simulink library "THAMO_6x2"  (R2018a)
settings: Solver=VariableStepAuto  StartTime=0.0  StopTime=10.0  RelTol=1e-3
undefined symbols (not defined in the file): BM, DiameterLastPiece, DPConstant, DPLinear, DPQuadratic, GeodeticHeight, ID, magnitude, MassFlow, Pressure, Temperature, Water
libraries: carnot x11, simulink x10, $bdroot x3
(part 3 of 3)

== system THAMO_6x2/Ventil/pressuredrop ==
  mdot : Inport
  p_in : Inport  Port=2
  clq_in : Inport  Port=3
  qua : Inport  Port=4
  Constant : Constant
  Constant1 : Constant  Value=0
  Constant2 : Constant  Value=0
  Dot Product : DotProduct  InputSameDT=on  OutDataTypeStr=Inherit: Inherit via internal rule
  Math Function : Math  Operator=square  SaturateOnIntegerOverflow=on
  Mux : Mux  Inputs=3
  Mux1 : Mux  Inputs=3
  Saturation : Saturate  UpperLimit=inf  LowerLimit=0
  sum : Sum  SaturateOnIntegerOverflow=on  InputSameDT=on  OutDataTypeStr=Inherit: Same as first input
  sum1 : Sum  Inputs=+-  SaturateOnIntegerOverflow=on  InputSameDT=on  OutDataTypeStr=Inherit: Same as first input
  p_out : Outport
  clq_out : Outport  Port=2
  wires:
  Saturation/1 -> p_out/1
  Constant/1 -> Mux/1
  mdot/1 -> Mux/2, Math Function/1
  Math Function/1 -> Mux/3
  Mux/1 -> Dot Product/1
  qua/1 -> Mux1/3
  clq_in/1 -> sum/1
  sum/1 -> clq_out/1
  Mux1/1 -> sum/2, Dot Product/2
  Dot Product/1 -> sum1/2
  p_in/1 -> sum1/1
  sum1/1 -> Saturation/1
  Constant1/1 -> Mux1/1
  Constant2/1 -> Mux1/2

== system THAMO_6x2/Verbraucher_RK-Modell/HK_MST_Ruehrkesselkask ==
  THB__1_W : Inport
  t__L : Inport  Port=2
  Bus Selector : BusSelector  OutputSignals=Temperature,MassFlow
  Bus Selector1 : BusSelector  OutputSignals=Temperature
  Constant1 : Constant  Value=t_1N
  Constant2 : Constant  Value=20
  Constant3 : Constant  Value=t_2N
  Mux : Mux  Inputs=3
  Subsystem : Subsystem
  THB_set_T : carnot/Source/Simple/THB_set_T
  cp : Lookup_n-D  NumberOfTableDimensions=1  BreakpointsForDimension1=[0,10,20,30,40,50,60,70,80,90,100]  Table=[4218,4192,4182,4179,4179,4181,4184,4190,4196,4205,4216]  InternalRulePriority=Speed  RndMeth=Simplest  InputSameDT=on
  dtlogN : Fcn  Expr=(u(1)-u(2))/log((u(1)-u(3))/(u(2)-u(3)))
  THB__2_W : Outport
  Qdot_2 : Outport  Port=2
  wires:
  Bus Selector1/1 -> cp/1  "<Temperature>"
  cp/1 -> Subsystem/4(cp)
  Subsystem/2(Qdot_he_w) -> Qdot_2/1  "Q_MST"
  Subsystem/1(T_he_out) -> THB_set_T/2  "T_RL_MST"
  dtlogN/1 -> Subsystem/5(dTlogN)
  THB__1_W/1 -> THB_set_T/1, Bus Selector/1, Bus Selector1/1
  THB_set_T/1 -> THB__2_W/1
  Bus Selector/2 -> Subsystem/2(mdot_w)  "<MassFlow>"
  Bus Selector/1 -> Subsystem/1(T_he_in)  "<Temperature>"
  t__L/1 -> Subsystem/3(T_i)
  Constant1/1 -> Mux/1
  Constant3/1 -> Mux/2
  Constant2/1 -> Mux/3
  Mux/1 -> dtlogN/1

== system THAMO_6x2/Verbraucher_RK-Modell/Pressure_Drop ==
  THB__1_W : Inport
  Bus Assignment1 : BusAssignment  AssignedSignals=Pressure,DPConstant,DPLinear,DPQuadratic
  Bus Selector3 : BusSelector  OutputSignals=MassFlow,Pressure
  Bus Selector4 : BusSelector  OutputSignals=DPConstant,DPLinear,DPQuadratic  OutputAsBus=on
  Bus Selector5 : BusSelector  OutputSignals=ID
  Compare To Constant1 : simulink/Logic and Bit Operations/Compare To Constant  relop=>  const=0  OutDataTypeStr=boolean
  Demux2 : Demux  Outputs=3
  Pressuredrop : carnot/Basic/Pressure_Drop/Pressuredrop
  lq_calc : Subsystem
  THB__2_W : Outport
  wires:
  Compare To Constant1/1 -> lq_calc/Enable
  lq_calc/1(qua) -> Pressuredrop/4
  Demux2/3 -> Bus Assignment1/5
  Demux2/2 -> Bus Assignment1/4
  Demux2/1 -> Bus Assignment1/3
  Bus Assignment1/1 -> THB__2_W/1
  Pressuredrop/1 -> Bus Assignment1/2
  THB__1_W/1 -> Bus Selector5/1, lq_calc/1(THB__1_W), Bus Selector4/1, Bus Selector3/1, Bus Assignment1/1
  Bus Selector4/1 -> Pressuredrop/3
  Bus Selector3/1 -> Pressuredrop/1  "<MassFlow>"
  Bus Selector3/2 -> Pressuredrop/2  "<Pressure>"
  Bus Selector5/1 -> Compare To Constant1/1  "<ID>"
  Pressuredrop/2 -> Demux2/1

== system THAMO_6x2/Wärmeabnehmer/Pressure_Drop ==
  THB__1_W : Inport
  Bus Assignment1 : BusAssignment  AssignedSignals=Pressure,DPConstant,DPLinear,DPQuadratic
  Bus Selector3 : BusSelector  OutputSignals=MassFlow,Pressure
  Bus Selector4 : BusSelector  OutputSignals=DPConstant,DPLinear,DPQuadratic  OutputAsBus=on
  Bus Selector5 : BusSelector  OutputSignals=ID
  Compare To Constant1 : simulink/Logic and Bit Operations/Compare To Constant  relop=>  const=0  OutDataTypeStr=boolean
  Demux2 : Demux  Outputs=3
  Pressuredrop : Subsystem  mask(pressure drop){}
      mask help:
      | Pressure drop according to input values of con, lin and qua:
      | dp = con + lin*mdot + qua*mdot²
      | The coefficients are also added to the correponding THB elements.
      mask Help: web(fullfile(path_carnot('help'),'Pressuredrop.html'),'-helpbrowser')
  lq_calc : Subsystem
  THB__2_W : Outport
  wires:
  Compare To Constant1/1 -> lq_calc/Enable
  lq_calc/1(qua) -> Pressuredrop/4(qua)
  Demux2/3 -> Bus Assignment1/5
  Demux2/2 -> Bus Assignment1/4
  Demux2/1 -> Bus Assignment1/3
  Bus Assignment1/1 -> THB__2_W/1
  Pressuredrop/1(p_out) -> Bus Assignment1/2
  THB__1_W/1 -> Bus Selector5/1, lq_calc/1(THB__1_W), Bus Selector4/1, Bus Selector3/1, Bus Assignment1/1
  Bus Selector4/1 -> Pressuredrop/3(clq_in)
  Bus Selector3/1 -> Pressuredrop/1(mdot)  "<MassFlow>"
  Bus Selector3/2 -> Pressuredrop/2(p_in)  "<Pressure>"
  Bus Selector5/1 -> Compare To Constant1/1  "<ID>"
  Pressuredrop/2(clq_out) -> Demux2/1

== system THAMO_6x2/Wärmeabnehmer/Temperatur ==
  THB__1_W : Inport
  Qdot_2 : Inport  Port=2
  Bus Assignment : BusAssignment  AssignedSignals=Temperature
  Bus Selector : BusSelector  OutputSignals=Temperature,MassFlow
  Fcn : Fcn  Expr=u(1)-u(4)/u(3)/u(2)
  Mux : Mux
  Thermal_Capacity : Subsystem  mask(Thermal Capacity){}
      mask help: Basic one node model of a thermal mass using the differential equation:
      mask Help: web(fullfile(path_carnot('help'),'Thermal_Capacity.html'),'-helpbrowser')
  cp_W : Lookup_n-D  NumberOfTableDimensions=1  BreakpointsForDimension1=[0,10,20,30,40,50,60,70,80,90,100]  Table=[4218,4192,4182,4179,4179,4181,4184,4190,4196,4205,4216]  InternalRulePriority=Speed  RndMeth=Simplest  InputSameDT=on
  THB__2_W : Outport
  wires:
  THB__1_W/1 -> Bus Assignment/1, Bus Selector/1
  Bus Assignment/1 -> Thermal_Capacity/1(THB__1_W)
  cp_W/1 -> Mux/3
  Bus Selector/2 -> Mux/2  "<MassFlow>"
  Bus Selector/1 -> cp_W/1, Mux/1  "<Temperature>"
  Qdot_2/1 -> Mux/4
  Mux/1 -> Fcn/1
  Fcn/1 -> Bus Assignment/2
  Thermal_Capacity/1(THB__2_W) -> THB__2_W/1

== system THAMO_6x2/Wärmeerzeuger/Pressure_Drop ==
  THB__1_W : Inport
  Bus Assignment1 : BusAssignment  AssignedSignals=Pressure,DPConstant,DPLinear,DPQuadratic
  Bus Selector3 : BusSelector  OutputSignals=MassFlow,Pressure
  Bus Selector4 : BusSelector  OutputSignals=DPConstant,DPLinear,DPQuadratic  OutputAsBus=on
  Bus Selector5 : BusSelector  OutputSignals=ID
  Compare To Constant1 : simulink/Logic and Bit Operations/Compare To Constant  relop=>  const=0  OutDataTypeStr=boolean
  Demux2 : Demux  Outputs=3
  Pressuredrop : carnot/Basic/Pressure_Drop/Pressuredrop
  lq_calc : Subsystem
  THB__2_W : Outport
  wires:
  Compare To Constant1/1 -> lq_calc/Enable
  lq_calc/1(qua) -> Pressuredrop/4
  Demux2/3 -> Bus Assignment1/5
  Demux2/2 -> Bus Assignment1/4
  Demux2/1 -> Bus Assignment1/3
  Bus Assignment1/1 -> THB__2_W/1
  Pressuredrop/1 -> Bus Assignment1/2
  THB__1_W/1 -> Bus Selector5/1, lq_calc/1(THB__1_W), Bus Selector4/1, Bus Selector3/1, Bus Assignment1/1
  Bus Selector4/1 -> Pressuredrop/3
  Bus Selector3/1 -> Pressuredrop/1  "<MassFlow>"
  Bus Selector3/2 -> Pressuredrop/2  "<Pressure>"
  Bus Selector5/1 -> Compare To Constant1/1  "<ID>"
  Pressuredrop/2 -> Demux2/1

== system THAMO_6x2/Wärmeerzeuger/Thermal_Capacity ==
  mdot : Inport
  Tin : Inport  Port=2
  Divide : Product  Inputs=*/
  Integrator : Integrator  InitialCondition=Tamb
  Losses : Gain  Gain=UV  SaturateOnIntegerOverflow=on  OutDataTypeStr=Inherit: Same as input  ParamDataTypeStr=Inherit: Same as input
  Product1 : Product  Inputs=3  SaturateOnIntegerOverflow=on  InputSameDT=on  OutDataTypeStr=Inherit: Same as first input
  Product3 : Product  Inputs=3  SaturateOnIntegerOverflow=on  InputSameDT=on  OutDataTypeStr=Inherit: Same as first input
  Sum1 : Sum  Inputs=-+  SaturateOnIntegerOverflow=on  InputSameDT=on  OutDataTypeStr=Inherit: Same as first input
  Sum2 : Sum  Inputs=-+  SaturateOnIntegerOverflow=on  InputSameDT=on  OutDataTypeStr=Inherit: Same as first input
  Sum3 : Sum  Inputs=+-  SaturateOnIntegerOverflow=on  InputSameDT=on  OutDataTypeStr=Inherit: Same as first input
  Tamb : Constant  Value=Tamb
  Tamb1 : Constant  Value=V/1000
  cp : Lookup_n-D  NumberOfTableDimensions=1  BreakpointsForDimension1=[0,10,20,30,40,50,60,70,80,90,100]  Table=[4218,4192,4182,4179,4179,4181,4184,4190,4196,4205,4216]  InternalRulePriority=Speed  RndMeth=Simplest  InputSameDT=on
  rho : Lookup_n-D  NumberOfTableDimensions=1  BreakpointsForDimension1=[0,10,20,30,40,50,60,70,80,90,100]  Table=[999.84,999.7,998.2,995.64,992.21,988.03,983.19,977.76,971.79,965.3,958.35]  InternalRulePriority=Speed  RndMeth=Simplest  InputSameDT=on
  Tout : Outport
  wires:
  mdot/1 -> Product1/2
  Product1/1 -> Sum2/2
  Sum2/1 -> Divide/1
  Tamb/1 -> Sum3/2
  Losses/1 -> Sum2/1
  Sum3/1 -> Losses/1
  cp/1 -> Product3/1, Product1/3
  Divide/1 -> Integrator/1
  Sum1/1 -> Product1/1
  Tin/1 -> Sum1/2
  Product3/1 -> Divide/2
  rho/1 -> Product3/2
  Tamb1/1 -> Product3/3
  Integrator/1 -> rho/1, cp/1, Sum1/1, Sum3/1, Tout/1

== system THAMO_6x2/Überströmventil/pressuredrop ==
  mdot : Inport
  p_in : Inport  Port=2
  clq_in : Inport  Port=3
  con : Inport  Port=4
  lin : Inport  Port=5
  qua : Inport  Port=6
  Constant : Constant
  Dot Product : DotProduct  InputSameDT=on  OutDataTypeStr=Inherit: Inherit via internal rule
  Math Function : Math  Operator=square  SaturateOnIntegerOverflow=on
  Mux : Mux  Inputs=3
  Mux1 : Mux  Inputs=3
  Saturation : Saturate  UpperLimit=inf  LowerLimit=0
  sum : Sum  SaturateOnIntegerOverflow=on  InputSameDT=on  OutDataTypeStr=Inherit: Same as first input
  sum1 : Sum  Inputs=+-  SaturateOnIntegerOverflow=on  InputSameDT=on  OutDataTypeStr=Inherit: Same as first input
  p_out : Outport
  clq_out : Outport  Port=2
  wires:
  lin/1 -> Mux1/2
  con/1 -> Mux1/1
  sum1/1 -> Saturation/1
  p_in/1 -> sum1/1
  Dot Product/1 -> sum1/2
  Mux1/1 -> Dot Product/2, sum/2
  sum/1 -> clq_out/1
  clq_in/1 -> sum/1
  qua/1 -> Mux1/3
  Mux/1 -> Dot Product/1
  Math Function/1 -> Mux/3
  mdot/1 -> Math Function/1, Mux/2
  Constant/1 -> Mux/1
  Saturation/1 -> p_out/1

== system THAMO_6x2/Brennwertkessel/Combustion_Calculation/cp___A ==
  eco : Inport
  Add : Sum  Inputs=+++++++
  Add1 : Sum  Inputs=+++++++
  Bus Selector1 : BusSelector  OutputSignals=mdotH20,mdotCO2,mdot_O2,mdotSO2,mdotN2,mdotNOx,mdot_CO
  Divide : Product  Inputs=/*
  Product{,1..6} (7 alike) : Product
  cpCO : Constant  Value=1.04
  cpCO2 : Constant  Value=0.846
  cpH2O : Constant  Value=1.85
  cpN2 : Constant  Value=1.04
  cpNOx : Constant  Value=1.009
  cpO2 : Constant  Value=0.912
  cpSO2 : Constant  Value=0.632
  cp___A : Outport
  wires:
  Add/1 -> Divide/1
  Add1/1 -> Divide/2
  Divide/1 -> cp___A/1
  Product1/1 -> Add1/2
  Product2/1 -> Add1/3
  Product3/1 -> Add1/4
  Product4/1 -> Add1/5
  Product5/1 -> Add1/6
  Product/1 -> Add1/1
  Product6/1 -> Add1/7
  cpCO2/1 -> Product1/2
  cpO2/1 -> Product2/2
  cpSO2/1 -> Product3/2
  cpN2/1 -> Product4/2
  cpNOx/1 -> Product5/2
  cpCO/1 -> Product6/2
  cpH2O/1 -> Product/2
  Bus Selector1/7 -> Add/7, Product6/1  "<mdot_CO>"
  Bus Selector1/1 -> Add/1, Product/1  "<mdotH20>"
  Bus Selector1/2 -> Add/2, Product1/1  "<mdotCO2>"
  Bus Selector1/3 -> Add/3, Product2/1  "<mdot_O2>"
  Bus Selector1/4 -> Add/4, Product3/1  "<mdotSO2>"
  Bus Selector1/6 -> Add/6, Product5/1  "<mdotNOx>"
  Bus Selector1/5 -> Add/5, Product4/1  "<mdotN2>"
  eco/1 -> Bus Selector1/1

== system THAMO_6x2/Brennwertkessel/Combustion_Calculation/exhaust gas ==
  h : Inport
  c : Inport  Port=2
  s : Inport  Port=3
  n : Inport  Port=4
  w : Inport  Port=5
  Mux : Mux  Inputs=2
  kgCO2 : Gain  Gain=44.01/12  SaturateOnIntegerOverflow=on  OutDataTypeStr=Inherit: Same as input  ParamDataTypeStr=Inherit: Same as input
  kgH2O : Fcn  Expr=(18.01/1.008/2)*u(1)+u(2)
  kgN2 : Gain  Gain=0.5  SaturateOnIntegerOverflow=on  OutDataTypeStr=Inherit: Same as input  ParamDataTypeStr=Inherit: Same as input
  kgSO2 : Gain  Gain=64.06/32.06  SaturateOnIntegerOverflow=on  OutDataTypeStr=Inherit: Same as input  ParamDataTypeStr=Inherit: Same as input
  H2O : Outport
  CO2 : Outport  Port=2
  SO2 : Outport  Port=3
  N2 : Outport  Port=4
  wires:
  n/1 -> kgN2/1
  kgSO2/1 -> SO2/1
  kgH2O/1 -> H2O/1
  kgCO2/1 -> CO2/1
  Mux/1 -> kgH2O/1
  c/1 -> kgCO2/1
  h/1 -> Mux/1
  w/1 -> Mux/2
  s/1 -> kgSO2/1
  kgN2/1 -> N2/1

== system THAMO_6x2/Brennwertkessel/Pressure_Drop/lq_calc ==
  THB__1_W : Inport
  Enable : EnablePort
  Bus Selector1 : BusSelector  OutputSignals=Temperature,MassFlow
  Constant : Constant  Value=BM
  Constant1 : Constant  Value=kvs
  Constant2 : Constant  Value=zeta
  Constant3 : Constant  Value=d
  Constant4 : Constant  Value=m_N
  Constant5 : Constant  Value=dp_N
  Multiport Switch : MultiPortSwitch
  Mux : Mux  Inputs=2
  Mux1 : Mux  Inputs=2
  Mux2 : Mux
  calc_qua_N : Fcn  Expr=u(2)/u(1)^2
  calc_qua_kvs : Fcn  Expr=(3600^2*100)/(u(1)^2*u(2))
  calc_qua_zeta : Fcn  Expr=(((u(3)/u(1))/(3.1415/4*(u(4)/1000)^2))^2*u(2)*u(1)/2)/u(3)^2
  rho : Lookup_n-D  NumberOfTableDimensions=1  BreakpointsForDimension1=[0,10,20,30,40,50,60,70,80,90,100]  Table=[999.84,999.7,998.2,995.64,992.21,988.03,983.19,977.76,971.79,965.3,958.35]  InternalRulePriority=Speed  RndMeth=Simplest  InputSameDT=on
  qua : Outport
  wires:
  calc_qua_zeta/1 -> Multiport Switch/3
  Constant2/1 -> Mux2/2
  Mux2/1 -> calc_qua_zeta/1
  Bus Selector1/2 -> Mux2/3  "<MassFlow>"
  Constant3/1 -> Mux2/4
  calc_qua_N/1 -> Multiport Switch/4
  Constant5/1 -> Mux1/2
  Constant4/1 -> Mux1/1
  Mux1/1 -> calc_qua_N/1
  calc_qua_kvs/1 -> Multiport Switch/2
  Mux/1 -> calc_qua_kvs/1
  rho/1 -> Mux/2, Mux2/1
  Constant1/1 -> Mux/1
  Constant/1 -> Multiport Switch/1
  Multiport Switch/1 -> qua/1
  THB__1_W/1 -> Bus Selector1/1
  Bus Selector1/1 -> rho/1  "<Temperature>"

== system THAMO_6x2/Mischer/Ventil/Ventilkennlinie ==
  St : Inport
  THB__1_W : Inport  Port=2
  Bus Selector : BusSelector  OutputSignals=Temperature
  Constant2 : Constant  Value=ART
  Constant6 : Constant  Value=n_0
  Constant8 : Constant  Value=kvs
  GLP : Fcn  Expr=u(2)*((1/u(2))^u(1))
  Mux : Mux  Inputs=2
  Mux2 : Mux  Inputs=2
  Mux3 : Mux  Inputs=2
  Product : Product
  Switch : Switch  Criteria=u2 > Threshold  Threshold=1
  calc_qua_kvs : Fcn  Expr=(3600^2*100)/(u(1)^2*u(2))
  linear : Fcn  Expr=u(2)+(1-u(2))*u(1)
  rho : Lookup_n-D  NumberOfTableDimensions=1  BreakpointsForDimension1=[0,10,20,30,40,50,60,70,80,90,100]  Table=[999.84,999.7,998.2,995.64,992.21,988.03,983.19,977.76,971.79,965.3,958.35]  InternalRulePriority=Speed  RndMeth=Simplest  InputSameDT=on
  qua : Outport
  wires:
  rho/1 -> Mux/2
  Product/1 -> Mux/1
  Mux/1 -> calc_qua_kvs/1
  calc_qua_kvs/1 -> qua/1
  THB__1_W/1 -> Bus Selector/1
  GLP/1 -> Switch/1
  Constant2/1 -> Switch/2
  Switch/1 -> Product/1
  Constant8/1 -> Product/2
  Constant6/1 -> Mux3/2, Mux2/2
  Mux3/1 -> linear/1
  Mux2/1 -> GLP/1
  linear/1 -> Switch/3
  St/1 -> Mux3/1, Mux2/1
  Bus Selector/1 -> rho/1  "<Temperature>"

== system THAMO_6x2/Mischer/Ventil/pressuredrop ==
  mdot : Inport
  p_in : Inport  Port=2
  clq_in : Inport  Port=3
  qua : Inport  Port=4
  Constant : Constant
  Constant1 : Constant  Value=0
  Constant2 : Constant  Value=0
  Dot Product : DotProduct  InputSameDT=on  OutDataTypeStr=Inherit: Inherit via internal rule
  Math Function : Math  Operator=square  SaturateOnIntegerOverflow=on
  Mux : Mux  Inputs=3
  Mux1 : Mux  Inputs=3
  Saturation : Saturate  UpperLimit=inf  LowerLimit=0
  sum : Sum  SaturateOnIntegerOverflow=on  InputSameDT=on  OutDataTypeStr=Inherit: Same as first input
  sum1 : Sum  Inputs=+-  SaturateOnIntegerOverflow=on  InputSameDT=on  OutDataTypeStr=Inherit: Same as first input
  p_out : Outport
  clq_out : Outport  Port=2
  wires:
  Constant2/1 -> Mux1/2
  Constant1/1 -> Mux1/1
  sum1/1 -> Saturation/1
  p_in/1 -> sum1/1
  Dot Product/1 -> sum1/2
  Mux1/1 -> Dot Product/2, sum/2
  sum/1 -> clq_out/1
  clq_in/1 -> sum/1
  qua/1 -> Mux1/3
  Mux/1 -> Dot Product/1
  Math Function/1 -> Mux/3
  mdot/1 -> Math Function/1, Mux/2
  Constant/1 -> Mux/1
  Saturation/1 -> p_out/1

== system THAMO_6x2/Mischer/Ventil1/Ventilkennlinie ==
  St : Inport
  THB__1_W : Inport  Port=2
  Bus Selector : BusSelector  OutputSignals=Temperature
  Constant2 : Constant  Value=ART
  Constant6 : Constant  Value=n_0
  Constant8 : Constant  Value=kvs
  GLP : Fcn  Expr=u(2)*((1/u(2))^u(1))
  Mux : Mux  Inputs=2
  Mux2 : Mux  Inputs=2
  Mux3 : Mux  Inputs=2
  Product : Product
  Switch : Switch  Criteria=u2 > Threshold  Threshold=1
  calc_qua_kvs : Fcn  Expr=(3600^2*100)/(u(1)^2*u(2))
  linear : Fcn  Expr=u(2)+(1-u(2))*u(1)
  rho : Lookup_n-D  NumberOfTableDimensions=1  BreakpointsForDimension1=[0,10,20,30,40,50,60,70,80,90,100]  Table=[999.84,999.7,998.2,995.64,992.21,988.03,983.19,977.76,971.79,965.3,958.35]  InternalRulePriority=Speed  RndMeth=Simplest  InputSameDT=on
  qua : Outport
  wires:
  rho/1 -> Mux/2
  Product/1 -> Mux/1
  Mux/1 -> calc_qua_kvs/1
  calc_qua_kvs/1 -> qua/1
  THB__1_W/1 -> Bus Selector/1
  GLP/1 -> Switch/1
  Constant2/1 -> Switch/2
  Switch/1 -> Product/1
  Constant8/1 -> Product/2
  Constant6/1 -> Mux3/2, Mux2/2
  Mux3/1 -> linear/1
  Mux2/1 -> GLP/1
  linear/1 -> Switch/3
  St/1 -> Mux3/1, Mux2/1
  Bus Selector/1 -> rho/1  "<Temperature>"

== system THAMO_6x2/Mischer/Ventil1/pressuredrop ==
  mdot : Inport
  p_in : Inport  Port=2
  clq_in : Inport  Port=3
  qua : Inport  Port=4
  Constant : Constant
  Constant1 : Constant  Value=0
  Constant2 : Constant  Value=0
  Dot Product : DotProduct  InputSameDT=on  OutDataTypeStr=Inherit: Inherit via internal rule
  Math Function : Math  Operator=square  SaturateOnIntegerOverflow=on
  Mux : Mux  Inputs=3
  Mux1 : Mux  Inputs=3
  Saturation : Saturate  UpperLimit=inf  LowerLimit=0
  sum : Sum  SaturateOnIntegerOverflow=on  InputSameDT=on  OutDataTypeStr=Inherit: Same as first input
  sum1 : Sum  Inputs=+-  SaturateOnIntegerOverflow=on  InputSameDT=on  OutDataTypeStr=Inherit: Same as first input
  p_out : Outport
  clq_out : Outport  Port=2
  wires:
  Constant2/1 -> Mux1/2
  Constant1/1 -> Mux1/1
  sum1/1 -> Saturation/1
  p_in/1 -> sum1/1
  Dot Product/1 -> sum1/2
  Mux1/1 -> Dot Product/2, sum/2
  sum/1 -> clq_out/1
  clq_in/1 -> sum/1
  qua/1 -> Mux1/3
  Mux/1 -> Dot Product/1
  Math Function/1 -> Mux/3
  mdot/1 -> Math Function/1, Mux/2
  Constant/1 -> Mux/1
  Saturation/1 -> p_out/1

== system THAMO_6x2/Rohr/Druckverlust/Pressuredrop ==
  mdot : Inport
  p_in : Inport  Port=2
  clq_in : Inport  Port=3
  con : Inport  Port=4
  lin : Inport  Port=5
  qua : Inport  Port=6
  Constant : Constant
  Dot Product : DotProduct  InputSameDT=on  OutDataTypeStr=Inherit: Inherit via internal rule
  Math Function : Math  Operator=square  SaturateOnIntegerOverflow=on
  Mux : Mux  Inputs=3
  Mux1 : Mux  Inputs=3
  Saturation : Saturate  UpperLimit=inf  LowerLimit=0
  sum : Sum  SaturateOnIntegerOverflow=on  InputSameDT=on  OutDataTypeStr=Inherit: Same as first input
  sum1 : Sum  Inputs=+-  SaturateOnIntegerOverflow=on  InputSameDT=on  OutDataTypeStr=Inherit: Same as first input
  p_out : Outport
  clq_out : Outport  Port=2
  wires:
  Saturation/1 -> p_out/1
  Constant/1 -> Mux/1
  mdot/1 -> Mux/2, Math Function/1
  Math Function/1 -> Mux/3
  Mux/1 -> Dot Product/1
  con/1 -> Mux1/1
  lin/1 -> Mux1/2
  qua/1 -> Mux1/3
  clq_in/1 -> sum/1
  sum/1 -> clq_out/1
  Mux1/1 -> sum/2, Dot Product/2
  Dot Product/1 -> sum1/2
  p_in/1 -> sum1/1
  sum1/1 -> Saturation/1

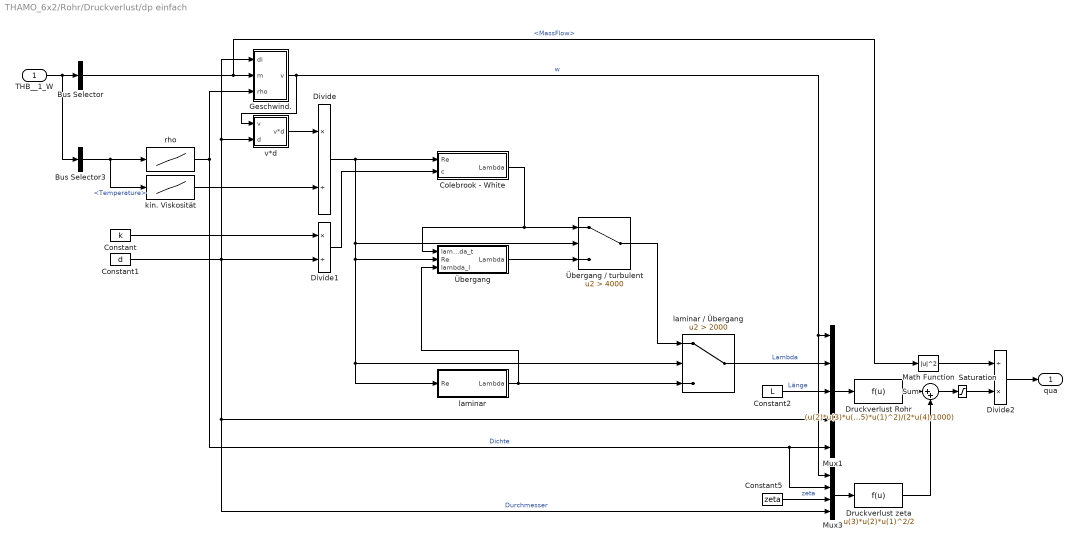
== system THAMO_6x2/Rohr/Druckverlust/dp einfach ==
  THB__1_W : Inport
  Bus Selector : BusSelector  OutputSignals=MassFlow
  Bus Selector3 : BusSelector  OutputSignals=Temperature
  Colebrook - White : Subsystem
  Constant : Constant  Value=k
  Constant1 : Constant  Value=d
  Constant2 : Constant  Value=L
  Constant5 : Constant  Value=zeta
  Divide : Product  Inputs=*/
  Divide1 : Product  Inputs=*/
  Divide2 : Product  Inputs=/*
  Druckverlust Rohr : Fcn  Expr=(u(2)*u(3)*u(5)*u(1)^2)/(2*u(4)/1000)
  Druckverlust zeta : Fcn  Expr=u(3)*u(2)*u(1)^2/2
  Geschwind. : Subsystem
  Math Function : Math  Operator=magnitude^2  SaturateOnIntegerOverflow=on
  Mux1 : Mux  Inputs=5
  Mux3 : Mux
  Saturation : Saturate  UpperLimit=inf  LowerLimit=1
  Sum : Sum  Inputs=|++
  kin. Viskosität : Lookup_n-D  NumberOfTableDimensions=1  BreakpointsForDimension1=[1,10,20,30,40,50,60,70,80,90,99]  Table=[0.017307,0.013061,0.010033,0.0080078,0.0065808,0.0055346,0.0047437,0.0041308,0.0036464,0.0032572,0.0029690]/(100*100)  InternalRulePriority=Speed  RndMeth=Simplest  InputSameDT=on
  laminar : Subsystem
  laminar / Übergang : Switch  Criteria=u2 > Threshold  Threshold=2000
  rho : Lookup_n-D  NumberOfTableDimensions=1  BreakpointsForDimension1=[0,10,20,30,40,50,60,70,80,90,100]  Table=[999.84,999.7,998.2,995.64,992.21,988.03,983.19,977.76,971.79,965.3,958.35]  InternalRulePriority=Speed  RndMeth=Simplest  InputSameDT=on
  v*d : Subsystem
  Übergang : Subsystem
  Übergang / turbulent : Switch  Criteria=u2 > Threshold  Threshold=4000
  qua : Outport
  wires:
  v*d/1(v*d) -> Divide/1
  Constant/1 -> Divide1/1
  Divide1/1 -> Colebrook - White/2(c)
  laminar/1(Lambda) -> laminar / Übergang/3, Übergang/3(lambda_l)
  laminar / Übergang/1 -> Mux1/2  "Lambda"
  Constant2/1 -> Mux1/3  "Länge"
  Mux1/1 -> Druckverlust Rohr/1
  rho/1 -> Geschwind./3(rho), Mux3/2, Mux1/5  "Dichte"
  Geschwind./1(v) -> Mux3/1, Mux1/1, v*d/1(v)  "w"
  Divide/1 -> Übergang / turbulent/2, Übergang/2(Re), laminar/1(Re), laminar / Übergang/2, Colebrook - White/1(Re)
  THB__1_W/1 -> Bus Selector3/1, Bus Selector/1
  Übergang / turbulent/1 -> laminar / Übergang/1
  Colebrook - White/1(Lambda) -> Übergang / turbulent/1, Übergang/1(lambda_t)
  Übergang/1(Lambda) -> Übergang / turbulent/3
  Constant1/1 -> Mux3/4, Mux1/4, v*d/2(d), Geschwind./1(di), Divide1/2  "Durchmesser"
  Mux3/1 -> Druckverlust zeta/1
  Constant5/1 -> Mux3/3  "zeta"
  Bus Selector/1 -> Math Function/1, Geschwind./2(m)  "<MassFlow>"
  Druckverlust Rohr/1 -> Sum/1
  Druckverlust zeta/1 -> Sum/2
  Math Function/1 -> Divide2/1
  Sum/1 -> Saturation/1
  Divide2/1 -> qua/1
  Saturation/1 -> Divide2/2
  Bus Selector3/1 -> kin. Viskosität/1, rho/1  "<Temperature>"
  kin. Viskosität/1 -> Divide/2

== system THAMO_6x2/T-Stueck mischend/Mixer/Mix_T_Mdot ==
  THB1 : Inport
  THB2 : Inport  Port=2
  Bus Selector1 : BusSelector  OutputSignals=MassFlow,Temperature
  Bus Selector2 : BusSelector  OutputSignals=MassFlow,Temperature
  Fcn : Fcn  Expr=(u(1)*u(2)+u(3)*u(4))/(u(1)+u(3))
  Mux : Mux
  T : Outport
  wires:
  THB2/1 -> Bus Selector1/1
  THB1/1 -> Bus Selector2/1
  Bus Selector2/2 -> Mux/2  "<Temperature>"
  Bus Selector2/1 -> Mux/1  "<MassFlow>"
  Bus Selector1/1 -> Mux/3  "<MassFlow>"
  Bus Selector1/2 -> Mux/4  "<Temperature>"
  Mux/1 -> Fcn/1
  Fcn/1 -> T/1

== system THAMO_6x2/T-Stueck mischend/Mixer/decrease_ID1 ==
  In1 : Inport
  Abs : Abs
  Bias : Bias  Bias=-1
  Dot Product1 : DotProduct  InputSameDT=on  OutDataTypeStr=Inherit: Inherit via internal rule
  Sign : Signum
  Out1 : Outport
  wires:
  Bias/1 -> Dot Product1/2
  Sign/1 -> Dot Product1/1
  Abs/1 -> Bias/1
  Dot Product1/1 -> Out1/1
  In1/1 -> Sign/1, Abs/1

== system THAMO_6x2/T-Stueck mischend/Mixer/decrease_ID2 ==
  In1 : Inport
  Abs : Abs
  Bias : Bias  Bias=-1
  Dot Product1 : DotProduct  InputSameDT=on  OutDataTypeStr=Inherit: Inherit via internal rule
  Sign : Signum
  Out1 : Outport
  wires:
  In1/1 -> Abs/1, Sign/1
  Dot Product1/1 -> Out1/1
  Abs/1 -> Bias/1
  Sign/1 -> Dot Product1/1
  Bias/1 -> Dot Product1/2

== system THAMO_6x2/Verbraucher_RK-Modell/HK_MST_Ruehrkesselkask/Subsystem ==
  T_he_in : Inport
  mdot_w : Inport  Port=2
  T_i : Inport  Port=3
  cp : Inport  Port=4
  dTlogN : Inport  Port=5
  Constant1 : Constant  Value=Qdot_N
  Constant2 : Constant  Value=n
  K : Fcn  Expr=u(3)/(u(1)^n)
  Mux : Mux  Inputs=6
  Mux1 : Mux  Inputs=6
  Mux2 : Mux  Inputs=6
  Mux3 : Mux
  Mux4 : Mux  Inputs=3
  Qdot_he_w_ : Fcn  Expr=u(4)*u(2)*(u(1)-u(3))
  T_w1 : Integrator  InitialConditionSource=external
  T_w2 : Integrator  InitialConditionSource=external
  T_w3 : Integrator  InitialConditionSource=external
  dT_w1/dt : Fcn  Expr=(3*u(2)*u(5)*(u(3)-u(1))-u(6)*(u(1)-u(4))^n)/(M*u(5))
  dT_w2/dt : Fcn  Expr=(3*u(2)*u(5)*(u(3)-u(1))-u(6)*(u(1)-u(4))^n)/(M*u(5))
  dT_w3/dt : Fcn  Expr=(3*u(2)*u(5)*(u(3)-u(1))-u(6)*(u(1)-u(4))^n)/(M*u(5))
  T_he_out : Outport
  Qdot_he_w : Outport  Port=2
  wires:
  K/1 -> Mux1/6, Mux/6, Mux2/6
  cp/1 -> Mux/5, Mux1/5, Mux2/5, Mux3/4  "cp"
  Mux4/1 -> K/1
  Constant1/1 -> Mux4/3
  Constant2/1 -> Mux4/2
  dTlogN/1 -> Mux4/1
  Mux2/1 -> dT_w3/dt/1
  Mux3/1 -> Qdot_he_w_/1
  Mux1/1 -> dT_w2/dt/1
  Mux/1 -> dT_w1/dt/1
  T_w2/1 -> Mux2/3, Mux1/1
  T_he_in/1 -> Mux/3, Mux3/1  "T_VL"
  dT_w2/dt/1 -> T_w2/1
  Qdot_he_w_/1 -> Qdot_he_w/1
  T_w3/1 -> Mux2/1, Mux3/3, T_he_out/1  "T_RL"
  T_i/1 -> Mux/4, T_w1/2, Mux1/4, Mux2/4, T_w3/2, T_w2/2
  T_w1/1 -> Mux1/3, Mux/1
  dT_w3/dt/1 -> T_w3/1
  dT_w1/dt/1 -> T_w1/1
  mdot_w/1 -> Mux3/2, Mux/2, Mux1/2, Mux2/2  "mdot"

== system THAMO_6x2/Verbraucher_RK-Modell/Pressure_Drop/lq_calc ==
  THB__1_W : Inport
  Enable : EnablePort
  Bus Selector : BusSelector  OutputSignals=MassFlow
  Bus Selector1 : BusSelector  OutputSignals=Temperature
  Constant : Constant  Value=BM
  Constant1 : Constant  Value=kvs
  Constant2 : Constant  Value=zeta
  Constant3 : Constant  Value=d
  Constant4 : Constant  Value=m_N
  Constant5 : Constant  Value=dp_N
  Multiport Switch : MultiPortSwitch
  Mux : Mux  Inputs=2
  Mux1 : Mux  Inputs=2
  Mux2 : Mux
  calc_qua_N : Fcn  Expr=u(2)/u(1)^2
  calc_qua_kvs : Fcn  Expr=(3600^2*100)/(u(1)^2*u(2))
  calc_qua_zeta : Fcn  Expr=(((u(3)/u(1))/(3.1415/4*(u(4)/1000)^2))^2*u(2)*u(1)/2)/u(3)^2
  rho : Lookup_n-D  NumberOfTableDimensions=1  BreakpointsForDimension1=[0,10,20,30,40,50,60,70,80,90,100]  Table=[999.84,999.7,998.2,995.64,992.21,988.03,983.19,977.76,971.79,965.3,958.35]  InternalRulePriority=Speed  RndMeth=Simplest  InputSameDT=on
  qua : Outport
  wires:
  Bus Selector1/1 -> rho/1  "<Temperature>"
  calc_qua_zeta/1 -> Multiport Switch/3
  Constant2/1 -> Mux2/2
  Mux2/1 -> calc_qua_zeta/1
  Bus Selector/1 -> Mux2/3  "<MassFlow>"
  Constant3/1 -> Mux2/4
  calc_qua_N/1 -> Multiport Switch/4
  Constant5/1 -> Mux1/2
  Constant4/1 -> Mux1/1
  Mux1/1 -> calc_qua_N/1
  calc_qua_kvs/1 -> Multiport Switch/2
  Mux/1 -> calc_qua_kvs/1
  rho/1 -> Mux/2, Mux2/1
  Constant1/1 -> Mux/1
  Constant/1 -> Multiport Switch/1
  Multiport Switch/1 -> qua/1
  THB__1_W/1 -> Bus Selector/1, Bus Selector1/1

== system THAMO_6x2/Wärmeabnehmer/Pressure_Drop/Pressuredrop ==
  mdot : Inport
  p_in : Inport  Port=2
  clq_in : Inport  Port=3
  qua : Inport  Port=4
  Constant : Constant
  Constant1 : Constant  Value=0
  Constant2 : Constant  Value=0
  Dot Product : DotProduct  InputSameDT=on  OutDataTypeStr=Inherit: Inherit via internal rule
  Math Function : Math  Operator=square  SaturateOnIntegerOverflow=on
  Mux : Mux  Inputs=3
  Mux1 : Mux  Inputs=3
  Saturation : Saturate  UpperLimit=inf  LowerLimit=0
  sum : Sum  SaturateOnIntegerOverflow=on  InputSameDT=on  OutDataTypeStr=Inherit: Same as first input
  sum1 : Sum  Inputs=+-  SaturateOnIntegerOverflow=on  InputSameDT=on  OutDataTypeStr=Inherit: Same as first input
  p_out : Outport
  clq_out : Outport  Port=2
  wires:
  Saturation/1 -> p_out/1
  Constant/1 -> Mux/1
  mdot/1 -> Mux/2, Math Function/1
  Math Function/1 -> Mux/3
  Mux/1 -> Dot Product/1
  Constant1/1 -> Mux1/1
  Constant2/1 -> Mux1/2
  qua/1 -> Mux1/3
  clq_in/1 -> sum/1
  sum/1 -> clq_out/1
  Mux1/1 -> sum/2, Dot Product/2
  Dot Product/1 -> sum1/2
  p_in/1 -> sum1/1
  sum1/1 -> Saturation/1

== system THAMO_6x2/Wärmeabnehmer/Pressure_Drop/lq_calc ==
  THB__1_W : Inport
  Enable : EnablePort
  Bus Selector : BusSelector  OutputSignals=MassFlow
  Constant : Constant  Value=BM
  Constant1 : Constant  Value=kvs
  Constant2 : Constant  Value=zeta
  Constant3 : Constant  Value=d
  Constant4 : Constant  Value=m_N
  Constant5 : Constant  Value=dp_N
  Density : carnot/Basic/Material_Properties/Density  VariantControl=CarlibClassic  INPUTARGUMENTS=THB  DEBUGLEVEL=DEBUGLEVEL  MAXTOTALWARNINGS=inf  MAXCONSECUTIVEWARNINGS=inf  WRITETOFILE=0  FILENAME='errors.txt'
  Multiport Switch : MultiPortSwitch
  Mux : Mux  Inputs=2
  Mux1 : Mux  Inputs=2
  Mux2 : Mux
  calc_qua_N : Fcn  Expr=u(2)/u(1)^2
  calc_qua_kvs : Fcn  Expr=(3600^2*100)/(u(1)^2*u(2))
  calc_qua_zeta : Fcn  Expr=(((u(3)/u(1))/(3.1415/4*(u(4)/1000)^2))^2*u(2)*u(1)/2)/u(3)^2
  qua : Outport
  wires:
  calc_qua_zeta/1 -> Multiport Switch/3
  Constant2/1 -> Mux2/2
  Mux2/1 -> calc_qua_zeta/1
  Bus Selector/1 -> Mux2/3  "<MassFlow>"
  Constant3/1 -> Mux2/4
  calc_qua_N/1 -> Multiport Switch/4
  Constant5/1 -> Mux1/2
  Constant4/1 -> Mux1/1
  Mux1/1 -> calc_qua_N/1
  calc_qua_kvs/1 -> Multiport Switch/2
  Mux/1 -> calc_qua_kvs/1
  Density/1 -> Mux/2, Mux2/1
  Constant1/1 -> Mux/1
  Constant/1 -> Multiport Switch/1
  Multiport Switch/1 -> qua/1
  THB__1_W/1 -> Bus Selector/1, Density/1

== system THAMO_6x2/Wärmeabnehmer/Temperatur/Thermal_Capacity ==
  THB__1_W : Inport
  Bus Assignment : BusAssignment  AssignedSignals=Temperature
  Bus Selector : BusSelector  OutputSignals=Temperature,MassFlow
  Constant : Constant  Value=M
  Divide : Product  Inputs=*//
  Integrator : Integrator  InitialCondition=20
  Product1 : Product  Inputs=3  SaturateOnIntegerOverflow=on  InputSameDT=on  OutDataTypeStr=Inherit: Same as first input
  Sum1 : Sum  Inputs=-+  SaturateOnIntegerOverflow=on  InputSameDT=on  OutDataTypeStr=Inherit: Same as first input
  cp_W : Lookup_n-D  NumberOfTableDimensions=1  BreakpointsForDimension1=[0,10,20,30,40,50,60,70,80,90,100]  Table=[4218,4192,4182,4179,4179,4181,4184,4190,4196,4205,4216]  InternalRulePriority=Speed  RndMeth=Simplest  InputSameDT=on
  THB__2_W : Outport
  wires:
  Integrator/1 -> Sum1/1, Bus Assignment/2
  Product1/1 -> Divide/1
  cp_W/1 -> Divide/3, Product1/3
  Divide/1 -> Integrator/1
  Sum1/1 -> Product1/1
  THB__1_W/1 -> Bus Assignment/1, Bus Selector/1
  Bus Assignment/1 -> THB__2_W/1
  Bus Selector/1 -> cp_W/1, Sum1/2  "<Temperature>"
  Bus Selector/2 -> Product1/2  "<MassFlow>"
  Constant/1 -> Divide/2

== system THAMO_6x2/Wärmeerzeuger/Pressure_Drop/lq_calc ==
  THB__1_W : Inport
  Enable : EnablePort
  Bus Selector1 : BusSelector  OutputSignals=Temperature,MassFlow
  Constant : Constant  Value=BM
  Constant1 : Constant  Value=kvs
  Constant2 : Constant  Value=zeta
  Constant3 : Constant  Value=d
  Constant4 : Constant  Value=m_N
  Constant5 : Constant  Value=dp_N
  Multiport Switch : MultiPortSwitch
  Mux : Mux  Inputs=2
  Mux1 : Mux  Inputs=2
  Mux2 : Mux
  calc_qua_N : Fcn  Expr=u(2)/u(1)^2
  calc_qua_kvs : Fcn  Expr=(3600^2*100)/(u(1)^2*u(2))
  calc_qua_zeta : Fcn  Expr=(((u(3)/u(1))/(3.1415/4*(u(4)/1000)^2))^2*u(2)*u(1)/2)/u(3)^2
  rho : Lookup_n-D  NumberOfTableDimensions=1  BreakpointsForDimension1=[0,10,20,30,40,50,60,70,80,90,100]  Table=[999.84,999.7,998.2,995.64,992.21,988.03,983.19,977.76,971.79,965.3,958.35]  InternalRulePriority=Speed  RndMeth=Simplest  InputSameDT=on
  qua : Outport
  wires:
  calc_qua_zeta/1 -> Multiport Switch/3
  Constant2/1 -> Mux2/2
  Mux2/1 -> calc_qua_zeta/1
  Bus Selector1/2 -> Mux2/3  "<MassFlow>"
  Constant3/1 -> Mux2/4
  calc_qua_N/1 -> Multiport Switch/4
  Constant5/1 -> Mux1/2
  Constant4/1 -> Mux1/1
  Mux1/1 -> calc_qua_N/1
  calc_qua_kvs/1 -> Multiport Switch/2
  Mux/1 -> calc_qua_kvs/1
  rho/1 -> Mux/2, Mux2/1
  Constant1/1 -> Mux/1
  Constant/1 -> Multiport Switch/1
  Multiport Switch/1 -> qua/1
  THB__1_W/1 -> Bus Selector1/1
  Bus Selector1/1 -> rho/1  "<Temperature>"

== system THAMO_6x2/Rohr/Druckverlust/dp einfach/Colebrook - White ==
  Re : Inport
  c : Inport  Port=2
  Mux1 : Mux  Inputs=2
  turbulent : Fcn  Expr=0.25*(log10((5.74/(u(1)^0.9))+(u(2)/3.7)))^(-2)
  Lambda : Outport
  wires:
  c/1 -> Mux1/2
  Re/1 -> Mux1/1
  turbulent/1 -> Lambda/1
  Mux1/1 -> turbulent/1

== system THAMO_6x2/Rohr/Druckverlust/dp einfach/Geschwind. ==
  di : Inport
  m : Inport  Port=2
  rho : Inport  Port=3
  Fcn : Fcn  Expr=u(2)/u(3)/(((u(1)/1000)/2)^2*3.1415)
  Mux : Mux  Inputs=3
  v : Outport
  wires:
  di/1 -> Mux/1
  Mux/1 -> Fcn/1
  Fcn/1 -> v/1
  m/1 -> Mux/2
  rho/1 -> Mux/3

== system THAMO_6x2/Rohr/Druckverlust/dp einfach/laminar ==
  Re : Inport
  laminar : Fcn  Expr=64/u(1)
  Lambda : Outport
  wires:
  Re/1 -> laminar/1
  laminar/1 -> Lambda/1

== system THAMO_6x2/Rohr/Druckverlust/dp einfach/v*d ==
  v : Inport
  d : Inport  Port=2
  Fcn : Fcn  Expr=u(1)*u(2)/1000
  Mux : Mux  Inputs=2
  v*d : Outport
  wires:
  Mux/1 -> Fcn/1
  Fcn/1 -> v*d/1
  v/1 -> Mux/1
  d/1 -> Mux/2

== system THAMO_6x2/Rohr/Druckverlust/dp einfach/Übergang ==
  lambda_t : Inport
  Re : Inport  Port=2
  lambda_l : Inport  Port=3
  Mux1 : Mux  Inputs=3
  Übergang : Fcn  Expr=(u(1)-u(3))/2000*(u(2)-2000)+u(3)
  Lambda : Outport
  wires:
  lambda_l/1 -> Mux1/3
  lambda_t/1 -> Mux1/1
  Übergang/1 -> Lambda/1
  Mux1/1 -> Übergang/1
  Re/1 -> Mux1/2

== matlab function THAMO_6x2/Pumpenregelung/MATLAB Function ==
  data: St output; dp0 input; dp1 input; dp2 input; PUMP input; a0 input; a1 input; a2 input; Vp input; Vm input
function St = fcn(dp0,dp1,dp2,PUMP,a0,a1,a2,Vp,Vm)

if PUMP == 3
    mpu = max(roots([(dp2-a2) (dp1-a1) (dp0-a0)]));
    b   = max(roots([a2 a1 (a0-Vp)]));
    mpr = max(roots([dp2 dp1-(Vp/2)/b dp0-Vp/2]));
    if mpr > Vm
        St = real(mpr/mpu);
    else
        St = real(sqrt(((dp2*Vm^2+dp1*Vm+dp0)/(a2*Vm^2+a1*Vm+a0))));
    end
elseif PUMP == 2
    mkr = max(roots([dp2 dp1 (dp0-Vp)]));
    mku = max(roots([(dp2-a2) (dp1-a1) (dp0-a0)]));  
    if mkr > Vm
        St = real(mkr/mku);
    else
        St = real(sqrt(((dp2*Vm^2+dp1*Vm+dp0)/(a2*Vm^2+a1*Vm+a0))));
    end
else
    St = 1;
end

== matlab function THAMO_6x2/Haupt-Pumpe/Wirkungsgrad/MATLAB Function ==
  data: a0 input; a1 input; a2 input; eta output; eta_N input; a input; m input; St input
function eta = fcn(a0,a1,a2,eta_N,a,m,St)

eta_max = 1-(1-eta_N/100)*St^a; 
m_max = max(roots([a2 a1*St a0*St^2]));

eta = real(4*eta_max/m_max*(m-m^2/m_max));

end

== matlab function THAMO_6x2/Haupt-Pumpe/MATLAB Function ==
  data: a0 input; a1 input; a2 input; m output; dp0 input; dp1 input; dp2 input
function m = fcn(a0,a1,a2,dp0,dp1,dp2)
m =  real(max(roots([a2-dp2 a1-dp1 a0-dp0])));
end

== matlab function THAMO_6x2/Brennwertkessel/Wirkungsgrad ==
  data: t_2_A input; t_con input; WG output; hw input; bw input; WG_WEhw input; t_hw_A input
function WG = fcn(t_2_A,t_con,hw,bw,WG_WEhw,t_hw_A)

Kon = 1-(622*(611.2*exp(17.62*t_2_A/(243.12+t_2_A))))/(101300-(611.2*exp(17.62*t_2_A/(243.12+t_2_A))))/(622*(611.2*exp(17.62*t_con/(243.12+t_con))/(101300-(611.2*exp(17.62*t_con/(243.12+t_con))))));

if Kon < 0
    WG_con = 0;
else
    WG_con = Kon;
end

if t_2_A < t_con
    Avl = 0;
else
    Avl = WG_WEhw/(t_hw_A-t_con)*(t_2_A-t_con);
end

if t_2_A < t_con
    WG = 1+WG_con*bw/hw-WG_con;
else
    WG = 1-Avl;
end

== matlab function THAMO_6x2/3-Punkt-Regler/TVL-Regler nach t_a ==
  data: TVL_SOLL output; t_a input; TVLmax input; TVLmin input; T_HG input
function TVL_SOLL = fcn(t_a,TVLmax,TVLmin, T_HG)

m = (TVLmin-TVLmax)/(T_HG+16); 
TVL_SOLL = m*(t_a+16)+TVLmax;

== matlab function THAMO_6x2/Regler mit Fernfühler ohne mmin-Überwachung/TVL-Regler nach t_a ==
  data: TVL_SOLL output; t_a input; TVLmax input; TVLmin input; T_HG input
function TVL_SOLL = fcn(t_a,TVLmax,TVLmin, T_HG)

m = (TVLmin-TVLmax)/(T_HG+16); 
TVL_SOLL = m*(t_a+16)+TVLmax;

== matlab function THAMO_6x2/Stufenloser Regler/TVL-Regler nach t_a ==
  data: TVL_SOLL output; t_a input; TVLmax input; TVLmin input; T_HG input
function TVL_SOLL = fcn(t_a,TVLmax,TVLmin, T_HG)

m = (TVLmin-TVLmax)/(T_HG+16); 
TVL_SOLL = m*(t_a+16)+TVLmax;

== matlab function THAMO_6x2/Wärmeerzeuger/Wirkungsgrad ==
  data: t_2_A input; t_con input; WG output; hw input; bw input; WG_WEhw input; t_hw_A input
function WG = fcn(t_2_A,t_con,hw,bw,WG_WEhw,t_hw_A)

Kon = 1-(622*(611.2*exp(17.62*t_2_A/(243.12+t_2_A))))/(101300-(611.2*exp(17.62*t_2_A/(243.12+t_2_A))))/(622*(611.2*exp(17.62*t_con/(243.12+t_con))/(101300-(611.2*exp(17.62*t_con/(243.12+t_con))))));

if Kon < 0
    WG_con = 0;
else
    WG_con = Kon;
end

if t_2_A < t_con
    Avl = 0;
else
    Avl = WG_WEhw/(t_hw_A-t_con)*(t_2_A-t_con);
end

if t_2_A < t_con
    WG = 1+WG_con*bw/hw-WG_con;
else
    WG = 1-Avl;
end

== matlab function THAMO_6x2/T-Stueck mischend/Mixer/Druckverlustkoeffizienten aus Fit-Funktion ==
  data: m_ist input; q1 input; c output; l1 input; c1 input; q2 input; l2 input; c2 input; l output; q output; fdiv output
function [c,l,q,fdiv]= fcn(m_ist,q1,l1,c1,q2,l2,c2)

A = [q1 l1 c1 q2 l2 c2]; 

%% Bestimmung des Stranges mit cmax, dieser ist dann immer Strang 2 (q2,l2,c2)
% Strang 1 (q1,l1,c1) ist ab hier immer der mit dem geringeren konstanten Koeffizienten c
cmax = max(c1,c2);
if cmax == c1
    q1 = A(4);
    l1 = A(5);
    c1 = A(6);
    q2 = A(1);  
    l2 = A(2);
    c2 = A(3);
    div = 0;
    cmin = 2;
else
    q1 = A(1);
    l1 = A(2);
    c1 = A(3);
    q2 = A(4);  
    l2 = A(5);
    c2 = A(6);
    div = 1;
    cmin = 1;
end

%% Anlegen von Arrays
dp1     = [linspace(0,c2*0.9,10) linspace(c2*0.9,c2*1.1,100) linspace(c2*1.1,2*10^5,10)];
dp_p    = [];
m_p     = [];
m1      = zeros(1,length(dp1));
m2      = zeros(1,length(dp1));

%% Erzeugung der Anlagenkennlinien von Strang 1, Strang 2 und gesamt
for i=1:length(dp1)
    m1(i) = max(real(roots([q1 l1 c1-dp1(i)])));
    m2(i) = max(real(roots([q2 l2 c2-dp1(i)])));
end
mg_g = m1+m2; 

%% Berechnung des passenden qlc-Satzes für die Gesamtkennlinie
% Unter Berücksichtgung einer nicht stetigen Gesamtkennlinie 
if q1*m_ist^2+l1*m_ist+c1 >= c2
    for i = 1:length(dp1)
        if dp1(i) >= c2
            dp_p = [dp_p dp1(i)];
            m_p  = [m_p mg_g(i)];
        end
    end
    qlc = polyfit(m_p,dp_p,2); 
    q = qlc(1);
    l = qlc(2);
    c = qlc(3);
    dp_ist = q*m_ist^2+l*m_ist+c;
    if cmin == 1
        m1_ist = max(real(roots([q1 l1 c1-dp_ist])));
    else
        m1_ist = max(real(roots([q2 l2 c2-dp_ist])));
    end
    fdiv = m1_ist/m_ist;
else
    q = q1;
    l = l1;
    c = c1;
    fdiv = div;
end

== matlab function THAMO_6x2/TVL-Regler mit Hysterese/TVL-Regler nach t_a ==
  data: TVL_SOLL output; t_a input; TVLmax input; TVLmin input; T_HG input
function TVL_SOLL = fcn(t_a,TVLmax,TVLmin, T_HG)

m = (TVLmin-TVLmax)/(T_HG+16); 
TVL_SOLL = m*(t_a+16)+TVLmax;
